simulink model "Redresseur_MLI_3Ph_dq_model_boucle_de_tension_PLL"  (R2018b)
settings: Solver=ode8  StartTime=0.0  StopTime=Ts  FixedStep=1e-6  RelTol=1e-3
undefined symbols (not defined in the file): C, Im, inverter_matrix, K, Kpll, Kt, L, Q, R, Req, Td, Ti, Tipll, Tit, V, w, wf
libraries: simulink x3, simulink_extras x2, powerlib_meascontrol x1, powerlib x1
settings Model: Creator=driss  LastModifiedBy=driss
settings DataIOCC: ReturnWorkspaceOutputs=on
settings DebuggingCC: UnconnectedInputMsg=none  UnconnectedOutputMsg=none  UnconnectedLineMsg=none
settings ModelReferenceCC: EnableRefExpFcnMdlSchedulingChecks=off
settings RTWCC: Description=Generic Real-Time Target

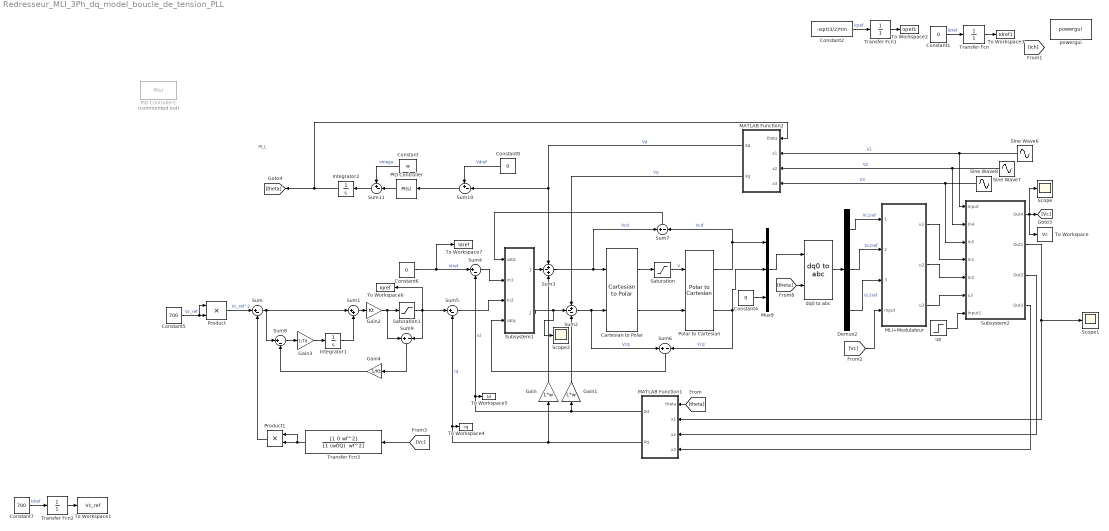
== system Redresseur_MLI_3Ph_dq_model_boucle_de_tension_PLL ==
  note: PLL
  Cartesian to Polar : simulink_extras/Transformations/Cartesian to Polar
      settings: SourceProductName=Simulink
  Constant : Constant  Value=w
  Constant{1,4,6,8} (4 alike) : Constant  Value=0
  Constant2 : Constant  Value=-sqrt(3/2)*Im
  Constant5 : Constant  Value=700
  Constant7 : Constant  Value=700
  Demux2 : Demux  Outputs=3
  Gain : Gain  Gain=L*w
  Gain1 : Gain  Gain=L*w
  Gain2 : Gain  Gain=Kt
  Gain3 : Gain  Gain=1/Tit
  Gain4 : Gain  Gain=1/Kt
  Integrator1 : Integrator
  Integrator2 : Integrator
  MATLAB Function1 : MATLAB Function  TreatAsAtomicUnit=on
  MATLAB Function2 : MATLAB Function  TreatAsAtomicUnit=on
  MLI+Modulateur : Subsystem
  Mux9 : Mux  Inputs=3
  PID Controller : simulink/Continuous/PID Controller  Controller=PI  Form=Parallel  TimeDomain=Continuous-time  SampleTime=-1  IntegratorMethod=Forward Euler  FilterMethod=Forward Euler  ControllerParametersSource=internal  P=Kpll  I=1/Tipll  D=0  UseFilter=on  N=100  TunerSelectOption=Transfer Function Based (PID Tuner App)  InitialConditionSource=internal  InitialConditionForIntegrator=0  InitialConditionForFilter=0  DifferentiatorICPrevScaledInput=0  ExternalReset=none  TrackingMode=off  Kt=1  LimitOutput=off  UpperSaturationLimit=inf  LowerSaturationLimit=-inf  LinearizeAsGain=on  AntiWindupMode=none  Kb=1  POutMin=[]  POutMax=[]  IOutMin=[]  IOutMax=[]  DOutMin=[]  DOutMax=[]  NOutMin=[]  NOutMax=[]  SumOutMin=[]  SumOutMax=[]  SaturationOutMin=[]  SaturationOutMax=[]  PParamMin=[]  PParamMax=[]  IParamMin=[]  IParamMax=[]  DParamMin=[]  DParamMax=[]  NParamMin=[]  NParamMax=[]  KbParamMin=[]  KbParamMax=[]  KtParamMin=[]  KtParamMax=[]  KbOutMin=[]  KbOutMax=[]  KtOutMin=[]  KtOutMax=[]  IntegratorOutMin=[]  IntegratorOutMax=[]  FilterOutMin=[]  FilterOutMax=[]  SumI1OutMin=[]  SumI1OutMax=[]  SumI2OutMin=[]  SumI2OutMax=[]  SumI3OutMin=[]  SumI3OutMax=[]  SumI4OutMin=[]  SumI4OutMax=[]  SumDOutMin=[]  SumDOutMax=[]  DifferentiatorOutMin=[]  DifferentiatorOutMax=[]  FilterDiffOutCoefMin=[]  FilterDiffOutCoefMax=[]  ReciprocalOutMin=[]  ReciprocalOutMax=[]  SumDenOutMin=[]  SumDenOutMax=[]  SumNumOutMin=[]  SumNumOutMax=[]  DivideOutMin=[]  DivideOutMax=[]  IntegratorContinuousStateAttributes=''  IntegratorStateMustResolveToSignalObject=off  IntegratorRTWStateStorageClass=Auto  FilterContinuousStateAttributes=''  FilterStateMustResolveToSignalObject=off  FilterRTWStateStorageClass=Auto  ParallelPVariant=InternalParameters  IdealPVariant=Disabled  IVariant=InternalParameters  DVariant=Disabled  IntegratorVariant=Continuous  SatVariant=Disabled  AWVariant=Passthrough  PCopyVariant=Disabled  TRVariant=Disabled  FdbkBlocksVariant=Forward  IdealPFdbkVariant=Disabled  SatFdbkVariant=Disabled  DerivativeFilterVariant=Disabled  NVariant=Disabled  NCopyVariant=Disabled_SignalSpec  FilterICVariant=Disabled  IntegratorICVariant=InternalICs  ExternalResetVariant=Disabled  TRSumVariant=Passthrough  SumFdbkVariant=Disabled  SumVariant=Sum_PI
  PID Controller1 : simulink/Continuous/PID Controller  Commented=on  Controller=PI  Form=Parallel  TimeDomain=Continuous-time  SampleTime=-1  IntegratorMethod=Forward Euler  FilterMethod=Forward Euler  ControllerParametersSource=internal  P=Kt  I=1/Tit  D=0  UseFilter=on  N=100  TunerSelectOption=Transfer Function Based (PID Tuner App)  InitialConditionSource=internal  InitialConditionForIntegrator=0  InitialConditionForFilter=0  DifferentiatorICPrevScaledInput=0  ExternalReset=none  TrackingMode=off  Kt=1  LimitOutput=off  UpperSaturationLimit=inf  LowerSaturationLimit=-inf  LinearizeAsGain=on  AntiWindupMode=none  Kb=1  POutMin=[]  POutMax=[]  IOutMin=[]  IOutMax=[]  DOutMin=[]  DOutMax=[]  NOutMin=[]  NOutMax=[]  SumOutMin=[]  SumOutMax=[]  SaturationOutMin=[]  SaturationOutMax=[]  PParamMin=[]  PParamMax=[]  IParamMin=[]  IParamMax=[]  DParamMin=[]  DParamMax=[]  NParamMin=[]  NParamMax=[]  KbParamMin=[]  KbParamMax=[]  KtParamMin=[]  KtParamMax=[]  KbOutMin=[]  KbOutMax=[]  KtOutMin=[]  KtOutMax=[]  IntegratorOutMin=[]  IntegratorOutMax=[]  FilterOutMin=[]  FilterOutMax=[]  SumI1OutMin=[]  SumI1OutMax=[]  SumI2OutMin=[]  SumI2OutMax=[]  SumI3OutMin=[]  SumI3OutMax=[]  SumI4OutMin=[]  SumI4OutMax=[]  SumDOutMin=[]  SumDOutMax=[]  DifferentiatorOutMin=[]  DifferentiatorOutMax=[]  FilterDiffOutCoefMin=[]  FilterDiffOutCoefMax=[]  ReciprocalOutMin=[]  ReciprocalOutMax=[]  SumDenOutMin=[]  SumDenOutMax=[]  SumNumOutMin=[]  SumNumOutMax=[]  DivideOutMin=[]  DivideOutMax=[]  IntegratorContinuousStateAttributes=''  IntegratorStateMustResolveToSignalObject=off  IntegratorRTWStateStorageClass=Auto  FilterContinuousStateAttributes=''  FilterStateMustResolveToSignalObject=off  FilterRTWStateStorageClass=Auto  ParallelPVariant=InternalParameters  IdealPVariant=Disabled  IVariant=InternalParameters  DVariant=Disabled  IntegratorVariant=Continuous  SatVariant=Disabled  AWVariant=Passthrough  PCopyVariant=Disabled  TRVariant=Disabled  FdbkBlocksVariant=Forward  IdealPFdbkVariant=Disabled  SatFdbkVariant=Disabled  DerivativeFilterVariant=Disabled  NVariant=Disabled  NCopyVariant=Disabled_SignalSpec  FilterICVariant=Disabled  IntegratorICVariant=InternalICs  ExternalResetVariant=Disabled  TRSumVariant=Passthrough  SumFdbkVariant=Disabled  SumVariant=Sum_PI
  Polar to Cartesian : simulink_extras/Transformations/Polar to Cartesian
      settings: SourceProductName=Simulink  SourceProductBaseCode=SL
  Product : Product
  Product1 : Product
  Saturation : Saturate  UpperLimit=381  LowerLimit=0
  Saturation1 : Saturate  UpperLimit=0  LowerLimit=-sqrt(3/2)*Im
  Scope : Scope
  Scope1 : Scope
  Scope2 : Scope
  Sine Wave6 : Sin  Amplitude=V*sqrt(2)  Frequency=2*50*pi  SampleTime=0
  Sine Wave7 : Sin  Amplitude=V*sqrt(2)  Frequency=2*50*pi  Phase=-2*pi/3  SampleTime=0
  Sine Wave8 : Sin  Amplitude=V*sqrt(2)  Frequency=2*50*pi  Phase=-4*pi/3  SampleTime=0
  Subsystem1 : Subsystem
  Subsystem2 : Subsystem
  Sum{,4..5,8} (4 alike) : Sum  Inputs=|+-
  Sum1 : Sum  Inputs=|++
  Sum10 : Sum  Inputs=+-|
  Sum11 : Sum  Inputs=+-|
  Sum2 : Sum  Inputs=+--
  Sum3 : Sum  Inputs=+-+
  Sum6 : Sum  Inputs=+-
  Sum7 : Sum  Inputs=+-
  Sum9 : Sum  Inputs=+-
  To Workspace : ToWorkspace  VariableName=Vc  SaveFormat=Timeseries  SampleTime=-1
  To Workspace1 : ToWorkspace  VariableName=Vc_ref  SaveFormat=Timeseries  SampleTime=-1
  To Workspace2 : ToWorkspace  VariableName=Iqref1  SaveFormat=Timeseries  SampleTime=-1
  To Workspace3 : ToWorkspace  VariableName=Idref1  SaveFormat=Timeseries  SampleTime=-1
  To Workspace4 : ToWorkspace  VariableName=Iq  SaveFormat=Timeseries  SampleTime=-1
  To Workspace5 : ToWorkspace  VariableName=Id  SaveFormat=Timeseries  SampleTime=-1
  To Workspace6 : ToWorkspace  VariableName=Iqref  SaveFormat=Timeseries  SampleTime=-1
  To Workspace7 : ToWorkspace  VariableName=Idref  SaveFormat=Timeseries  SampleTime=-1
  Transfer Fcn : TransferFcn  Denominator=[1]
  Transfer Fcn1 : TransferFcn  Denominator=[1]
  Transfer Fcn2 : TransferFcn  Denominator=[1]
  Transfer Fcn3 : TransferFcn  Numerator=[1 0 wf^2]  Denominator="[1 (wf/Q)  wf^2]"
  dq0 to abc : powerlib_meascontrol/Transformations/dq0 to abc  Alignment=Aligned with phase A axis
  powergui : powerlib/powergui  Priority=1  SimulationMode=Continuous  SampleTime=50e-6  frequency=60  Iterations=50  frequencyindice=60  Pbase=100e6  ErrMax=1e-4  UnitsV=kV  UnitsW=MW  buscounter=0  FunctionMessages=off  echomessages=off  EnableUseOfTLC=off  CurrentSourceSwitches=off  DisableSnubberDevices=off  DisableRonSwitches=off  DisableVfSwitches=off  DisplayEquations=off  SolverType=Tustin/Backward Euler (TBE)  Interpol=off  ExternalGateDelay=off  methode=off  Ts=100  x0status=blocks  SPID=on  SwTol=0  HookPort=off  RestoreLinks=warning  ResistiveCurrentMeasurement=off  Frange=[0:2:500]  Ylog=off  Xlog=on  ShowGrid=off  save=off  variable=ZData  structure=0  ZoomFFT=off  StartTime=0.0  cycles=1  DisplayStyle=1  fundamental=60  FreqAxis=off  MaxFrequency=1000  frequencyindicesteady=1  RmsSteady=1  display=off
  "up " : Step  Time=0.05  Before=1  After=0  SampleTime=0
  wires:
  MLI+Modulateur/1(u1) -> Subsystem2/4(In1)
  MLI+Modulateur/2(u2) -> Subsystem2/5(In2)
  MLI+Modulateur/3(u3) -> Subsystem2/6(u3)
  Sine Wave7/1 -> MATLAB Function2/3(x2), Subsystem2/2(In4)  "V2"
  Sine Wave8/1 -> MATLAB Function2/4(x3), Subsystem2/3(In5)  "V3"
  Sine Wave6/1 -> MATLAB Function2/2(x1), Subsystem2/1(Input)  "V1"
  Subsystem2/1(Out4) -> Scope/1, [Vc], To Workspace/1
  Demux2/2 -> MLI+Modulateur/2(2)  "Vc2ref"
  Demux2/1 -> MLI+Modulateur/1(1)  "Vc1ref"
  Demux2/3 -> MLI+Modulateur/3(3)  "Vc3ref"
  Subsystem2/2(Out1) -> Scope1/1, MATLAB Function1/2(x1)
  Subsystem2/3(Out2) -> MATLAB Function1/3(x2)
  Subsystem2/4(Out3) -> MATLAB Function1/4(x3)
  MATLAB Function1/1(Xd) -> Sum4/2, To Workspace5/1, Gain1/1  "Id"
  MATLAB Function1/2(Xq) -> Sum5/2, To Workspace4/1, Gain/1  "Iq"
  MATLAB Function2/1(Xd) -> Sum10/2, Sum3/1  "Vd"
  Sum2/1 -> Sum6/1, Cartesian to Polar/2  "Vcq"
  MATLAB Function2/2(Xq) -> Sum2/1  "Vq"
  Subsystem1/2(2) -> Scope2/1, Sum2/2
  Subsystem1/1(1) -> Sum3/2
  Sum4/1 -> Subsystem1/2(In1)
  Sum5/1 -> Subsystem1/3(In2)
  [Vc] -> MLI+Modulateur/4(Input)
  Sum3/1 -> Sum7/1, Cartesian to Polar/1  "Vcd"
  Saturation/1 -> Polar to Cartesian/1  "V"
  Cartesian to Polar/1 -> Saturation/1
  Polar to Cartesian/2 -> Mux9/2, Sum6/2  "Vcq'"
  Polar to Cartesian/1 -> Sum7/2, Mux9/1  "Vcd'"
  Gain/1 -> Sum3/3
  Gain1/1 -> Sum2/3
  Cartesian to Polar/2 -> Polar to Cartesian/2
  Mux9/1 -> dq0 to abc/1
  dq0 to abc/1 -> Demux2/1
  [theta] -> dq0 to abc/2
  Constant4/1 -> Mux9/3
  Sum7/1 -> Subsystem1/1(satd)
  Sum6/1 -> Subsystem1/4(satq)
  Constant1/1 -> Transfer Fcn/1  "Idref"
  Transfer Fcn/1 -> To Workspace3/1
  Transfer Fcn1/1 -> To Workspace2/1
  Constant2/1 -> Transfer Fcn1/1  "Iqref"
  Constant7/1 -> Transfer Fcn2/1  "Idref"
  Transfer Fcn2/1 -> To Workspace1/1
  Sum8/1 -> Gain3/1
  Saturation1/1 -> Sum5/1, Sum9/2, To Workspace6/1
  Sum/1 -> Sum8/1, Sum1/1
  Sum1/1 -> Gain2/1
  Gain4/1 -> Sum8/2
  Integrator1/1 -> Sum1/2
  Sum9/1 -> Gain4/1
  Gain2/1 -> Sum9/1, Saturation1/1
  Gain3/1 -> Integrator1/1
  Constant6/1 -> To Workspace7/1, Sum4/1  "Idref"
  Constant8/1 -> Sum10/1  "Vdref"
  Sum10/1 -> PID Controller/1
  PID Controller/1 -> Sum11/2
  [theta] -> MATLAB Function1/1(theta)
  Sum11/1 -> Integrator2/1
  Integrator2/1 -> MATLAB Function2/1(theta), [theta]
  Constant/1 -> Sum11/1  "omega"
  "up "/1 -> Subsystem2/7(Input1)
  Product/1 -> Sum/1  "Vc_ref^2"
  Constant5/1 -> Product/1, Product/2  "Vc_ref"
  Product1/1 -> Sum/2
  [Vc] -> Transfer Fcn3/1
  Transfer Fcn3/1 -> Product1/1, Product1/2

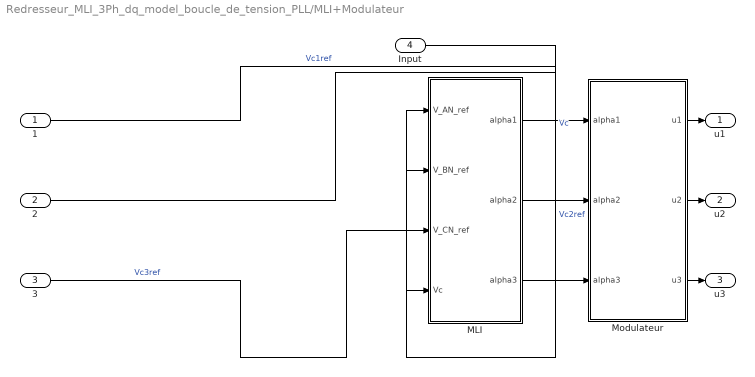
== system Redresseur_MLI_3Ph_dq_model_boucle_de_tension_PLL/MLI+Modulateur ==
  1 : Inport
  2 : Inport  Port=2
  3 : Inport  Port=3
  Input : Inport  Port=4
  MLI : Subsystem
  Modulateur : Subsystem
  u1 : Outport  VectorParamsAs1DForOutWhenUnconnected=on
  u2 : Outport  Port=2  VectorParamsAs1DForOutWhenUnconnected=on
  u3 : Outport  Port=3  VectorParamsAs1DForOutWhenUnconnected=on
  wires:
  MLI/3(alpha3) -> Modulateur/3(alpha3)
  Input/1 -> MLI/4(Vc)  "Vc"
  MLI/1(alpha1) -> Modulateur/1(alpha1)
  MLI/2(alpha2) -> Modulateur/2(alpha2)
  Modulateur/1(u1) -> u1/1
  Modulateur/2(u2) -> u2/1
  Modulateur/3(u3) -> u3/1
  3/1 -> MLI/3(V_CN_ref)  "Vc3ref"
  2/1 -> MLI/2(V_BN_ref)  "Vc2ref"
  1/1 -> MLI/1(V_AN_ref)  "Vc1ref"

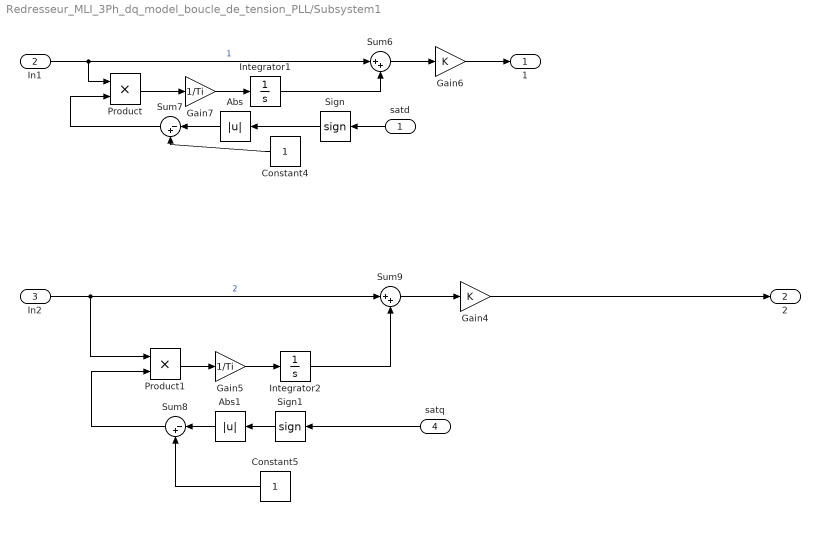
== system Redresseur_MLI_3Ph_dq_model_boucle_de_tension_PLL/Subsystem1 ==
  satd : Inport
  In1 : Inport  Port=2
  In2 : Inport  Port=3
  satq : Inport  Port=4
  Abs : Abs
  Abs1 : Abs
  Constant4 : Constant
  Constant5 : Constant
  Gain4 : Gain  Gain=K
  Gain5 : Gain  Gain=1/Ti
  Gain6 : Gain  Gain=K
  Gain7 : Gain  Gain=1/Ti
  Integrator1 : Integrator  InitialCondition=1
  Integrator2 : Integrator  InitialCondition=1
  Product : Product
  Product1 : Product
  Sign : Signum
  Sign1 : Signum
  Sum6 : Sum  Inputs=|++
  Sum7 : Sum  Inputs=|-+
  Sum8 : Sum  Inputs=|-+
  Sum9 : Sum  Inputs=|++
  1 : Outport  VectorParamsAs1DForOutWhenUnconnected=on
  2 : Outport  Port=2  VectorParamsAs1DForOutWhenUnconnected=on
  wires:
  Integrator2/1 -> Sum9/2
  Sign/1 -> Abs/1
  Sum7/1 -> Product/2
  In1/1 -> Sum6/1, Product/1  "1"
  Sum9/1 -> Gain4/1
  Abs/1 -> Sum7/1
  satq/1 -> Sign1/1
  Product1/1 -> Gain5/1
  Constant5/1 -> Sum8/2
  In2/1 -> Sum9/1, Product1/1  "2"
  Integrator1/1 -> Sum6/2
  Abs1/1 -> Sum8/1
  Gain7/1 -> Integrator1/1
  Constant4/1 -> Sum7/2
  Sum8/1 -> Product1/2
  Sum6/1 -> Gain6/1
  Gain5/1 -> Integrator2/1
  satd/1 -> Sign/1
  Product/1 -> Gain7/1
  Sign1/1 -> Abs1/1
  Gain6/1 -> 1/1
  Gain4/1 -> 2/1

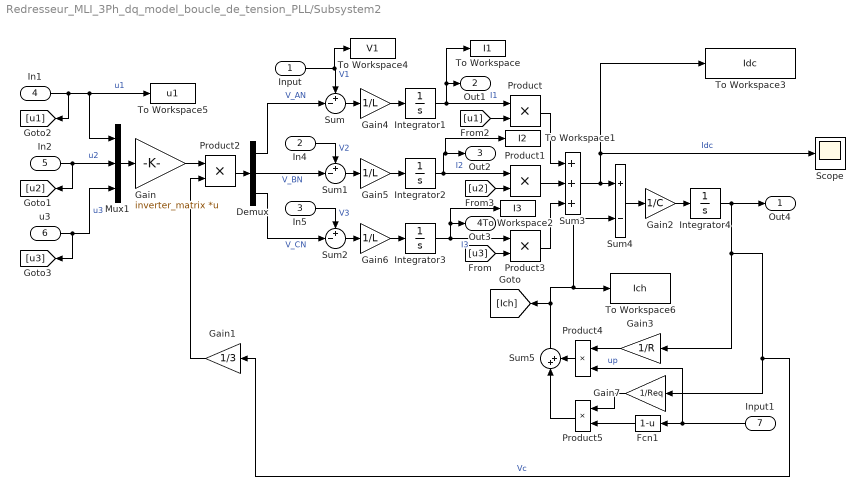
== system Redresseur_MLI_3Ph_dq_model_boucle_de_tension_PLL/Subsystem2 ==
  Input : Inport
  In4 : Inport  Port=2
  In5 : Inport  Port=3
  In1 : Inport  Port=4
  In2 : Inport  Port=5
  u3 : Inport  Port=6
  Input1 : Inport  Port=7
  Demux : Demux  Outputs=3
  Fcn1 : Fcn  Expr=1-u
  Gain : Gain  Gain=inverter_matrix  Multiplication=Matrix(K*u)
  Gain1 : Gain  Gain=1/3
  Gain2 : Gain  Gain=1/C
  Gain3 : Gain  Gain=1/R
  Gain4 : Gain  Gain=1/L
  Gain5 : Gain  Gain=1/L
  Gain6 : Gain  Gain=1/L
  Gain7 : Gain  Gain=1/Req
  Integrator1 : Integrator
  Integrator2 : Integrator
  Integrator3 : Integrator
  Integrator4 : Integrator  InitialCondition=V*sqrt(2)*sqrt(3)
  Mux1 : Mux  Inputs=3
  Product{,1..5} (6 alike) : Product
  Scope : Scope
  Sum : Sum  Inputs=+-|
  Sum1 : Sum  Inputs=+-|
  Sum2 : Sum  Inputs=+-|
  Sum3 : Sum  Inputs=+++
  Sum4 : Sum  Inputs=+-
  Sum5 : Sum  Inputs=|++
  To Workspace : ToWorkspace  VariableName=I1  SaveFormat=Timeseries  SampleTime=-1
  To Workspace1 : ToWorkspace  VariableName=I2  SaveFormat=Timeseries  SampleTime=-1
  To Workspace2 : ToWorkspace  VariableName=I3  SaveFormat=Timeseries  SampleTime=-1
  To Workspace3 : ToWorkspace  VariableName=Idc  SaveFormat=Timeseries  SampleTime=-1
  To Workspace4 : ToWorkspace  VariableName=V1  SaveFormat=Timeseries  SampleTime=-1
  To Workspace5 : ToWorkspace  VariableName=u1  SaveFormat=Timeseries  SampleTime=-1
  To Workspace6 : ToWorkspace  VariableName=Ich  SaveFormat=Timeseries  SampleTime=-1
  Out4 : Outport  VectorParamsAs1DForOutWhenUnconnected=on
  Out1 : Outport  Port=2  VectorParamsAs1DForOutWhenUnconnected=on
  Out2 : Outport  Port=3  VectorParamsAs1DForOutWhenUnconnected=on
  Out3 : Outport  Port=4  VectorParamsAs1DForOutWhenUnconnected=on
  wires:
  [u2] -> Product1/2
  [u1] -> Product/2
  Product2/1 -> Demux/1
  Gain6/1 -> Integrator3/1
  Gain5/1 -> Integrator2/1
  Gain4/1 -> Integrator1/1
  Integrator4/1 -> Out4/1, Gain3/1, Gain1/1, Gain7/1  "Vc"
  Gain2/1 -> Integrator4/1
  Sum4/1 -> Gain2/1
  Sum3/1 -> Scope/1, To Workspace3/1, Sum4/1  "Idc"
  Gain/1 -> Product2/1
  Gain1/1 -> Product2/2
  Product3/1 -> Sum3/3
  Product1/1 -> Sum3/2
  Product/1 -> Sum3/1
  [u3] -> Product3/2
  Mux1/1 -> Gain/1
  Integrator2/1 -> Out2/1, To Workspace1/1, Product1/1  "I2"
  Integrator3/1 -> Product3/1, Out3/1, To Workspace2/1  "I3"
  Integrator1/1 -> Product/1, Out1/1, To Workspace/1  "I1"
  Sum2/1 -> Gain6/1
  Sum1/1 -> Gain5/1
  Sum/1 -> Gain4/1
  In5/1 -> Sum2/1  "V3"
  In4/1 -> Sum1/1  "V2"
  Input/1 -> To Workspace4/1, Sum/1  "V1"
  Demux/1 -> Sum/2  "V_AN"
  Demux/3 -> Sum2/2  "V_CN"
  Demux/2 -> Sum1/2  "V_BN"
  In1/1 -> To Workspace5/1, Mux1/1, [u1]  "u1"
  In2/1 -> Mux1/2, [u2]  "u2"
  u3/1 -> Mux1/3, [u3]  "u3"
  Gain3/1 -> Product4/1
  Gain7/1 -> Product5/1
  Input1/1 -> Fcn1/1, Product4/2  "up"
  Product5/1 -> Sum5/1
  Product4/1 -> Sum5/2
  Sum5/1 -> [Ich], Sum4/2, To Workspace6/1
  Fcn1/1 -> Product5/2

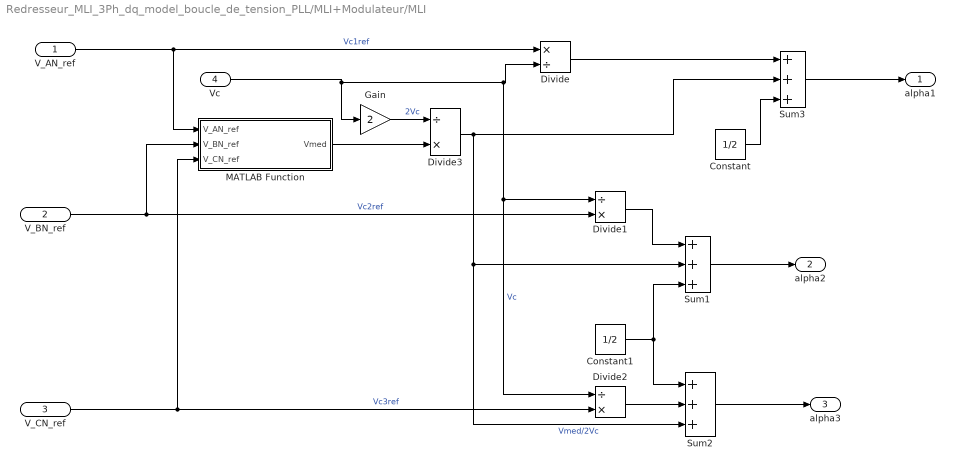
== system Redresseur_MLI_3Ph_dq_model_boucle_de_tension_PLL/MLI+Modulateur/MLI ==
  V_AN_ref : Inport
  V_BN_ref : Inport  Port=2
  V_CN_ref : Inport  Port=3
  Vc : Inport  Port=4
  Constant : Constant  Value=1/2
  Constant1 : Constant  Value=1/2
  Divide : Product  Inputs=*/
  Divide1 : Product  Inputs=/*
  Divide2 : Product  Inputs=/*
  Divide3 : Product  Inputs=/*
  Gain : Gain  Gain=2
  MATLAB Function : MATLAB Function  TreatAsAtomicUnit=on
  Sum1 : Sum  Inputs=+++
  Sum2 : Sum  Inputs=+++
  Sum3 : Sum  Inputs=+++
  alpha1 : Outport  VectorParamsAs1DForOutWhenUnconnected=on
  alpha2 : Outport  Port=2  VectorParamsAs1DForOutWhenUnconnected=on
  alpha3 : Outport  Port=3  VectorParamsAs1DForOutWhenUnconnected=on
  wires:
  Sum3/1 -> alpha1/1
  V_AN_ref/1 -> MATLAB Function/1(V_AN_ref), Divide/1  "Vc1ref"
  Divide/1 -> Sum3/1
  Constant/1 -> Sum3/3
  MATLAB Function/1(Vmed) -> Divide3/2
  Gain/1 -> Divide3/1  "2Vc"
  Constant1/1 -> Sum1/3, Sum2/1
  Sum1/1 -> alpha2/1
  Divide1/1 -> Sum1/1
  V_BN_ref/1 -> Divide1/2, MATLAB Function/2(V_BN_ref)  "Vc2ref"
  Divide3/1 -> Sum2/3, Sum1/2, Sum3/2  "Vmed/2Vc"
  Vc/1 -> Gain/1, Divide2/1, Divide1/1, Divide/2  "Vc"
  V_CN_ref/1 -> MATLAB Function/3(V_CN_ref), Divide2/2  "Vc3ref"
  Divide2/1 -> Sum2/2
  Sum2/1 -> alpha3/1

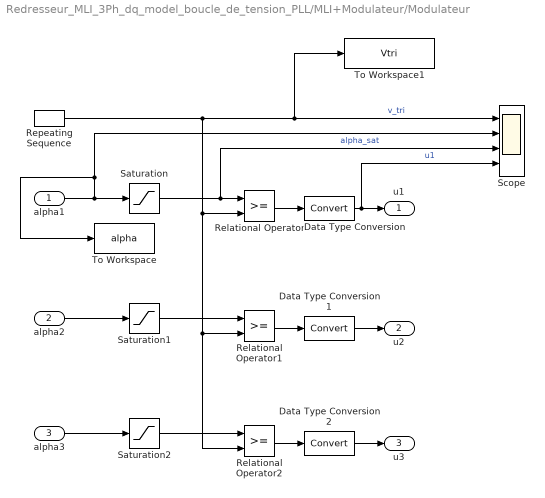
== system Redresseur_MLI_3Ph_dq_model_boucle_de_tension_PLL/MLI+Modulateur/Modulateur ==
  alpha1 : Inport
  alpha2 : Inport  Port=2
  alpha3 : Inport  Port=3
  Data Type Conversion : DataTypeConversion
  Data Type Conversion1 : DataTypeConversion
  Data Type Conversion2 : DataTypeConversion
  Relational Operator : RelationalOperator  OutDataTypeStr=boolean  RndMeth=Simplest
  Relational Operator1 : RelationalOperator  OutDataTypeStr=boolean  RndMeth=Simplest
  Relational Operator2 : RelationalOperator  OutDataTypeStr=boolean  RndMeth=Simplest
  Repeating Sequence : simulink/Sources/Repeating Sequence  rep_seq_t=[0 Td/2 Td]  rep_seq_y=[1 0 1]
  Saturation : Saturate  UpperLimit=1  LowerLimit=0
  Saturation1 : Saturate  UpperLimit=1  LowerLimit=0
  Saturation2 : Saturate  UpperLimit=1  LowerLimit=0
  Scope : Scope  NumInputPorts=4
  To Workspace : ToWorkspace  VariableName=alpha  SaveFormat=Timeseries  SampleTime=-1
  To Workspace1 : ToWorkspace  VariableName=Vtri  SaveFormat=Timeseries  SampleTime=-1
  u1 : Outport  VectorParamsAs1DForOutWhenUnconnected=on
  u2 : Outport  Port=2  VectorParamsAs1DForOutWhenUnconnected=on
  u3 : Outport  Port=3  VectorParamsAs1DForOutWhenUnconnected=on
  wires:
  Relational Operator/1 -> Data Type Conversion/1
  alpha1/1 -> To Workspace/1, Scope/2, Saturation/1
  Relational Operator1/1 -> Data Type Conversion1/1
  Relational Operator2/1 -> Data Type Conversion2/1
  Repeating Sequence/1 -> To Workspace1/1, Scope/1, Relational Operator1/2, Relational Operator2/2, Relational Operator/2  "v_tri"
  Saturation/1 -> Scope/3, Relational Operator/1  "alpha_sat"
  Data Type Conversion/1 -> u1/1, Scope/4  "u1"
  Data Type Conversion1/1 -> u2/1
  Data Type Conversion2/1 -> u3/1
  Saturation1/1 -> Relational Operator1/1
  alpha2/1 -> Saturation1/1
  alpha3/1 -> Saturation2/1
  Saturation2/1 -> Relational Operator2/1

== matlab function Redresseur_MLI_3Ph_dq_model_boucle_de_tension_PLL/MATLAB Function1 ==
  data: theta input; x1 input; Xd output; x2 input; x3 input; Xq output
function [Xd,Xq] = fcn(theta,x1,x2,x3)

Xd = sqrt(2/3)*(x1*cos(theta) + x2*cos(theta-2*pi/3) + x3*cos(theta+2*pi/3));
Xq = sqrt(2/3)*(-x1*sin(theta) - x2*sin(theta-2*pi/3) - x3*sin(theta+2*pi/3));

== matlab function Redresseur_MLI_3Ph_dq_model_boucle_de_tension_PLL/MLI+Modulateur/MLI/MATLAB Function ==
  data: V_AN_ref input; Vmed output; V_BN_ref input; V_CN_ref input
function Vmed = fcn(V_AN_ref,V_BN_ref,V_CN_ref)
     V_set = [V_AN_ref V_BN_ref V_CN_ref];
Vmed= -(min(V_set) + max(V_set));

== matlab function Redresseur_MLI_3Ph_dq_model_boucle_de_tension_PLL/MATLAB Function2 ==
  data: theta input; x1 input; Xd output; x2 input; x3 input; Xq output
function [Xd,Xq] = fcn(theta,x1,x2,x3)

Xd = sqrt(2/3)*(x1*cos(theta) + x2*cos(theta-2*pi/3) + x3*cos(theta+2*pi/3));
Xq = sqrt(2/3)*(-x1*sin(theta) - x2*sin(theta-2*pi/3) - x3*sin(theta+2*pi/3));
